simulink model "blockdemo"  (Simulink 6.3)
settings: Solver=FixedStepDiscrete  StartTime=0.0  StopTime=10.0  FixedStep=1  RelTol=1e-3
InitFcn:
  | %% DSPBuilder Start
  | alt_dspbuilder_update_model(bdroot)
  | %% DSPBuilder End
libraries: allblocks_alteradspbuilder2 x12
settings Model: LastModifiedBy=delphick

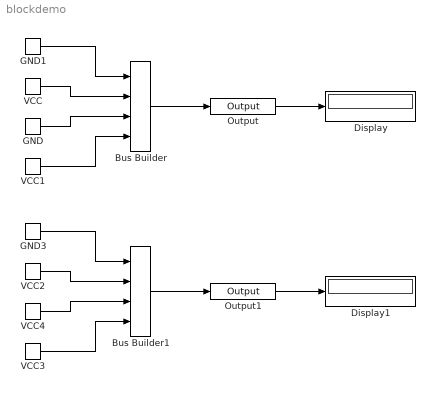
== system blockdemo ==
  Bus Builder : allblocks_alteradspbuilder2/Bus Builder  BusType=Signed Integer  bwl=4  bwr=1
  Bus Builder1 : allblocks_alteradspbuilder2/Bus Builder  BusType=Signed Integer  bwl=4  bwr=1
  Display : Display
  Display1 : Display
  GND : allblocks_alteradspbuilder2/GND  SpecifyClock=off
  GND1 : allblocks_alteradspbuilder2/GND  SpecifyClock=off
  GND3 : allblocks_alteradspbuilder2/GND  SpecifyClock=off
  Output : allblocks_alteradspbuilder2/Output  iofile=C:\workspace_clean\Documentation\DesignExamples\Tutorials\UnitBlocks\IOBus\GND_and_VCC\tb_blockdemo\blockdemo_Output.capture  BusType=Signed Integer  bwl=4  bwr=0  PORTTYPE=Output
  Output1 : allblocks_alteradspbuilder2/Output  iofile=C:\workspace_clean\Documentation\DesignExamples\Tutorials\UnitBlocks\IOBus\GND_and_VCC\tb_blockdemo\blockdemo_Output1.capture  BusType=Signed Integer  bwl=4  bwr=0  PORTTYPE=Output
  VCC{,1..4} (5 alike) : allblocks_alteradspbuilder2/VCC  SpecifyClock=off
  wires:
  Bus Builder/1 -> Output/1
  Output/1 -> Display/1
  GND1/1 -> Bus Builder/1
  VCC/1 -> Bus Builder/2
  GND/1 -> Bus Builder/3
  VCC1/1 -> Bus Builder/4
  Bus Builder1/1 -> Output1/1
  Output1/1 -> Display1/1
  GND3/1 -> Bus Builder1/1
  VCC2/1 -> Bus Builder1/2
  VCC4/1 -> Bus Builder1/3
  VCC3/1 -> Bus Builder1/4
